simulink model "kelvin_to_celsius_system"  (R2020b)
settings: Solver=VariableStepAuto  StartTime=0.0  StopTime=10.0  RelTol=1e-3
libraries: simulink x1
settings Model: PauseTimes=4  Creator=C-TEA  LastModifiedBy=C-TEA

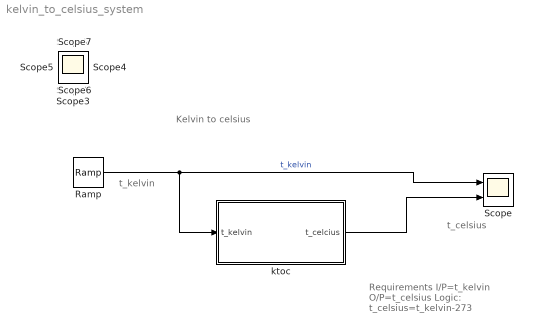
== system kelvin_to_celsius_system ==
  note: t_kelvin
  note: t_celsius
  note: Requirements
      | I/P=t_kelvin
      | O/P=t_celsius
      | Logic: t_celsius=t_kelvin-273
  note: Kelvin to celsius
  Ramp : simulink/Sources/Ramp  slope=1  start=20  InitialOutput=0
  Scope : Scope  NumInputPorts=2
  ktoc : Subsystem
  Scope{1..7} (7 alike) : Scope
  wires:
  Ramp/1 -> Scope/1, ktoc/1(t_kelvin)  "t_kelvin"
  ktoc/1(t_celcius) -> Scope/2

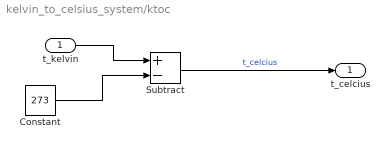
== system kelvin_to_celsius_system/ktoc ==
  t_kelvin : Inport
  Constant : Constant  Value=273
  Subtract : Sum  Inputs=+-
  t_celcius : Outport
  wires:
  Constant/1 -> Subtract/2
  t_kelvin/1 -> Subtract/1
  Subtract/1 -> t_celcius/1  "t_celcius"
